simulink model "testemplanner_cs"  (R2023a)
settings: Solver=ode5  StartTime=0.0  StopTime=70  FixedStep=1/1000  RelTol=1e-3
PreLoadFcn:
  | mbxruntime.callbacks.PreLoadFcn(bdroot);
PostLoadFcn:
  | mbxruntime.callbacks.PostLoadFcn(bdroot);
InitFcn:
  | mbxruntime.callbacks.InitFcn(bdroot);
StartFcn:
  | mbxruntime.callbacks.StartFcn(bdroot);
StopFcn:
  | mbxruntime.callbacks.StopFcn(bdroot);
model workspace (MAT data in the model file):
  mbox_table : object (value not decoded)
  model_closed = 0
  sim_status = 0
values from neighbouring files (symbols this model uses):
  c_factor = 43.75    [emplanner_init.m]
  cf = -175016    [emplanner_init.m]
  cr = -130634    [emplanner_init.m]
  global_path_x = [-4.4795 -3.48011774493 -2.48199463442 -1.48514775065 -0.489582877207 0.504698358082 1.49769585569 2.48941007764 3.47984169183 4.46899144113 5.45686009523 6.44344843293 ... (3001 elements, 3001x1)]    [global_path.mat]
  global_path_y = [6.0531 6.0531 6.0531 6.0531 6.0531 6.0531 6.0531 6.0531 6.0531 6.0531 6.0531 6.0531 ... (3001 elements, 3001x1)]    [global_path.mat]
  KD_PID_distance = 0.0    (= 0)    [emplanner_init.m]
  KD_PID_speed = 0    [emplanner_init.m]
  KI_PID_distance = 0.0    (= 0)    [emplanner_init.m]
  KI_PID_speed = 0    [emplanner_init.m]
  KP_PID_distance = 0.5    [emplanner_init.m]
  KP_PID_speed = 1.8    [emplanner_init.m]
  la = 1.265    [emplanner_init.m]
  lb = 2.947-1.265    (= 1.682)    [emplanner_init.m]
  LQR_K1 = k(:,1)'    [emplanner_init.m]
  LQR_K2 = k(:,2)'    [emplanner_init.m]
  LQR_K3 = k(:,3)'    [emplanner_init.m]
  LQR_K4 = k(:,4)'    [emplanner_init.m]
  m = 2020    [emplanner_init.m]
  rack_displacement = [-39.14 , -37.2 , -35.29 , -33.43 , -31.6 , -29.81 , -28.06 , -26.34 , -24.66 ,      -23.01 , -21.38 , -19.79 , -18.23 , -16.69 , -15.18 , -13.7 , -12.23 , -10.8 , -9.38 , -7.98 ,     -6.61 , -5.25 , -3.91 , -2.59 , -1.29 , 0 , 1.27 , 2.54 , 3.78 , 5.02 , 6.24 , 7.46 , 8.66 ,      9.86 , 11.05 , 12.24 , 13.41 , 14.59 , 15.76 , 16.92 , 18.09 , 19.25 , 20.42 , 21.59 , 22.76 ,      23.93 , 25.11 , 26 ...(+26 chars)    [emplanner_init.m]
  right_wheel_ground = [-70 ,-67.2 , -64.4 , -61.6 , -58.8 , -56 , -53.2 , -50.4 , -47.6 , -44.8 , -42 ,      -39.2 , -36.4 , -33.6 , -30.8 , -28 , -25.2 , -22.4 , -19.6 , -16.8 , -14 , -11.2 , -8.4 , -5.6 ,      -2.8 , 0 , 2.8 , 5.6 , 8.4 , 11.2 , 14 , 16.8 , 19.6 , 22.4 , 25.2 , 28 , 30.8 , 33.6 , 36.4 ,      39.2 , 42 , 44.8 , 47.6 , 50.4 , 53.2 , 56 , 58.8 , 61.6 , 64.4 , 67.2 , 70 ]    [emplanner_init.m]
  vx_break_point = zeros(1,5000)    [emplanner_init.m]
undefined symbols (not defined in the file or in its folder): aubr, DiscIntNeverNeededParam, tablebr, vubr, warningInitialVelocity, x0
libraries: PreScanSimulinkLibrary x19, simulink x19, simulink_extras x6, Solver_SF x1
(part 8 of 10)

== matlab function testemplanner_cs/Audi_A8_Sedan_1/decision&planning module/EM Planner/cacul planning start gcs ==
  data: pre_trajectory_x input; planning_start_x output; pre_trajectory_y input; pre_trajectory_heading input; pre_trajectory_kappa input; pre_trajectory_speed input; pre_trajectory_accel input; pre_trajectory_time input; current_time input; host_x input; host_y input; host_heading_xy input; host_vx input; host_vy input; host_ax input; host_ay input; planning_start_y output; planning_start_heading output; planning_start_kappa output; planning_start_vx output; planning_start_vy output; planning_start_ax output; planning_start_ay output; planning_start_time output; stitch_x output; stitch_y output; stitch_heading output; stitch_kappa output; stitch_speed output; stitch_accel output; stitch_time output
function [planning_start_x, planning_start_y, planning_start_heading, planning_start_kappa, planning_start_vx, ...
    planning_start_vy, planning_start_ax, planning_start_ay, planning_start_time, stitch_x, stitch_y, stitch_heading, stitch_kappa, ...
    stitch_speed, stitch_accel, stitch_time] = fcn(pre_trajectory_x, pre_trajectory_y, pre_trajectory_heading, ...
    pre_trajectory_kappa, pre_trajectory_speed,  pre_trajectory_accel, pre_trajectory_time, current_time, host_x, ...
    host_y, host_heading_xy, host_vx, host_vy, host_ax, host_ay)


%该模块用来计算规划起点的信息：x,y,heading,kappa,vx,vy,ax,ay
%以及待拼接的轨迹信息：stitch_x,y,heading,kappa...
%输入参数：hostx,y,heading,kappa是世界坐标系下，而vx,vy,ax,ay是基于车辆坐标系
%输出参数：规划开始点以及待拼接轨迹的vx,vy,ax,ay都是基于世界坐标系
%stitch用来存储规划起点前20个点的轨迹，要生成缓冲矩阵

stitch_x = zeros(20,1);
stitch_y = zeros(20,1);
stitch_heading = zeros(20,1);
stitch_kappa = zeros(20,1);
stitch_speed = zeros(20,1);
stitch_accel = zeros(20,1);
%待拼接矩阵的时间序列，用-1代表无需拼接
stitch_time = ones(20,1)*-1;

%定义持久变量，若是第一次运行...
%若不是第一次运行...
persistent is_first_run
if isempty(is_first_run)
    is_first_run = 0;
    %第一次运行时没有上一周期的规划结果，可以根据车辆运动学模型递推出current_time+100ms时的状态
    %但第一次运行时，没有初始车速、加速度，也不需要轨迹拼接，直接拿定位信息当作规划起点即可
    planning_start_x = host_x; 
    planning_start_y = host_y;
    planning_start_heading = host_heading_xy;
    planning_start_kappa = 0;
    %下面这一行是老王的写法，有疑问
    % planning_start_kappa = 0;
    planning_start_vx = 0;
    planning_start_vy = 0;
    planning_start_ax = 0;
    planning_start_ay = 0;
    %planning_start_time为规划起点对应的时间戳，而不是规划开始的时间
    planning_start_time = current_time+0.1;

else
    %若不是第一次运行
    %首先要在上周期规划的轨迹中寻找current所对应的索引的信息（应该处在什么位置），根据实际所处位置做出判断控制的效果、是否需要拼接轨迹及规划起点
    for i = 1:length(pre_trajectory_time)-1
        if pre_trajectory_time(i) <= current_time && pre_trajectory_time(i+1) > current_time
            break;
        end
    end
    %遍历出的i即为current_time所对应的序号
    %根据定位位置与理想位置之间的误差判断是否需要轨迹拼接
    x_current = host_x;
    y_current = host_y;   
    heading_current = host_heading_xy;
    %kappa_current = 0; %老王的写法，为什么现在的曲率是0？
    kappa_current = 0;
    %定位的vxvy...是基于车辆坐标系的，要转换成世界坐标系
    vx_current = host_vx*cos(heading_current)-host_vy*sin(heading_current);
    vy_current = host_vy*cos(heading_current)+host_vx*sin(heading_current);
    ax_current = host_ax*cos(heading_current)-host_ay*sin(heading_current);
    ay_current = host_ay*cos(heading_current)+host_ax*sin(heading_current);
    x_desire = pre_trajectory_x(i);
    y_desire = pre_trajectory_y(i);
    heading_desire = pre_trajectory_heading(i);
    tor1 = [cos(heading_desire); sin(heading_desire)];
    nor1 = [-sin(heading_desire); cos(heading_desire)];
    %根据误差向量及切向量和法向量计算定位和理想位置间的横向误差及纵向误差
    err_vector = [x_current; y_current]-[x_desire; y_desire];
    %纵向误差
    err_long = abs(err_vector'*tor1);
    %侧向误差
    err_lat = abs(err_vector'*nor1);
    %规划的周期是100ms，即0.1s
    dt = 0.1;
    %判断控制是否跟上了轨迹,一般认为纵向误差大于2或者横向误差大于0.5时控制效果差
    if err_long > 2.5 || err_lat > 0.5
        %控制没有跟上轨迹，需要根据车辆运动学模型递推一个周期得到规划起点的状态,这里认为车辆在一个周期内做匀加速直线运动
        planning_start_x = x_current+vx_current*dt+0.5*ax_current*dt^2;
        planning_start_y = y_current+vy_current*dt+0.5*ay_current*dt^2;
        
        planning_start_kappa = kappa_current;
        planning_start_vx = vx_current+ax_current*dt;
        planning_start_vy = vy_current+ay_current*dt;
        planning_start_heading = atan2(planning_start_vy,planning_start_vx);
        planning_start_ax = ax_current;
        planning_start_ay = ay_current;
        %把planning_start_time（规划开始时间）表述为current_time+0.1是否不妥，规划开始时间应为current_time,此处仍有疑问
        planning_start_time = current_time+0.1;
        %控制没有跟上规划，递推出下个周期规划起点后再拿上周期的规划结果做轨迹拼接也就没有意义
    else
        %控制跟上了规划，需要做轨迹拼接
        %规划起点是current_time+0.1在时间戳里对应的索引对应的信息
        %先找到规划起点的索引
        for j = i:length(pre_trajectory_time)-1
            if pre_trajectory_time(j) <= current_time+0.1 && pre_trajectory_time(j+1) > current_time+0.1
                break;
            end
        end
        %j即为current_time+0.1在pre_trajectory_time时间戳里的索引
        planning_start_x = pre_trajectory_x(j);
        planning_start_y = pre_trajectory_y(j);
        %pre_trajecctory_speed,accel为轨迹的切向速度、加速度
        planning_start_heading = pre_trajectory_heading(j);
        planning_start_kappa = pre_trajectory_kappa(j);
        planning_start_vx = pre_trajectory_speed(j)*cos(planning_start_heading);
        planning_start_vy = pre_trajectory_speed(j)*sin(planning_start_heading);
        %加速度分为切向加速度和法向加速度
        %计算规划起点的切向量和法向量
        tor2 = [cos(planning_start_heading); sin(planning_start_heading)];
        nor2 = [-sin(planning_start_heading); cos(planning_start_heading)];
        %计算规划起点的切向加速度和法向加速度
        a_tor = pre_trajectory_accel(j)*tor2;
        a_nor = pre_trajectory_speed(j)^2*planning_start_kappa*nor2;
        planning_start_ax = a_tor(1)+a_nor(1);
        planning_start_ay = a_tor(2)+a_nor(2);
        %下面的规划开始时间同样有疑问
        % planning_start_time = pre_trajectory_time(j);  
        planning_start_time = current_time+0.1;

        %下面开始准备轨迹拼接，分为规划起点之前足够20个点和不足20个点两种情况
        if j > 20
            stitch_x = pre_trajectory_x(j-20:j-1);
            stitch_y = pre_trajectory_y(j-20:j-1);
            stitch_heading = pre_trajectory_heading(j-20:j-1);
            stitch_kappa = pre_trajectory_kappa(j-20:j-1);
            stitch_speed = pre_trajectory_speed(j-20:j-1);
            stitch_accel = pre_trajectory_accel(j-20:j-1);
            stitch_time = pre_trajectory_time(j-20:j-1);
        else
            %q:如果j=1怎么办？
            %a：只要i！=j，j就不会为1；即current_time的索引不能等于current_time+0.1的索引
            %轨迹点的采样要足够密集；eg:如果1s采样一个点，则会i=j...
            stitch_x(22-j:20) = pre_trajectory_x(1:j-1);
            stitch_y(22-j:20) = pre_trajectory_y(1:j-1);
            stitch_heading(22-j:20) = pre_trajectory_heading(1:j-1);
            stitch_kappa(22-j:20) = pre_trajectory_kappa(1:j-1);
            stitch_speed(22-j:20) = pre_trajectory_speed(1:j-1);
            stitch_accel(22-j:20) = pre_trajectory_accel(1:j-1);
            stitch_time(22-j:20) = pre_trajectory_time(1:j-1);
        end
    end

end

== matlab function testemplanner_cs/Audi_A8_Sedan_1/decision&planning module/referenceline provider/MATLAB Function4 ==
  data: path_x input; path_heading output; path_y input; path_kappa output
function [path_heading, path_kappa] = fcn(path_x, path_y)

%原理：heading=atan(dy/dx)
%kappa=dheading/ds
%ds=(dx^2+dy^2)^0.5
%但角度存在多值性问题，例如heading=atan(dy/dx)=heading+pi,在三角函数运算时会出现问题
%可以容忍heading+2pi（三角函数运算不会出现问题），但计算kappa=(dheading+2pi)/ds时要做特殊处理
%很多奇怪问题的根源就是角度的多值性处理不当
%中点欧拉法不能直接用

%dx,dy而不是角度用中点欧拉
dx = diff(path_x);
dy = diff(path_y);

dx_pre = [dx(1);dx];
dx_end = [dx;dx(end)];
dx_final = (dx_pre+dx_end)/2;

dy_pre = [dy(1);dy];
dy_end = [dy;dy(end)];
dy_final = (dy_pre+dy_end)/2;

%.^2是对每一个元素做平方运算，^2是矩阵运算
ds_final = sqrt(dx_final.^2+dy_final.^2);

%atan2为四象限反正切，将角度限定在-pi-pi
path_heading = atan2(dy_final,dx_final);

%对heading做差分，得到dheading，同样采用中点欧拉
dheading = diff(path_heading);
dheading_pre = [dheading(1);dheading];
dheading_after = [dheading;dheading(end)];
dheading_final = (dheading_pre+dheading_after)/2;

%认为dheading为很小量，用sin(dheading)近似代替heading,因为sin(dheading)与sin(dheading+2pi)相等
path_kappa = dheading_final./ds_final;

== matlab function testemplanner_cs/Audi_A8_Sedan_1/decision&planning module/EM Planner/match&proj point search2 ==
  data: match_point_index_set output; proj_x_set output; proj_y_set output; proj_heading_set output; proj_kappa_set output; x_set input; y_set input; frenet_x_set input; frenet_y_set input; frenet_heading_set input; frenet_kapppa_set input
function [match_point_index_set, proj_x_set, proj_y_set, proj_heading_set, proj_kappa_set] = fcn(x_set, y_set, frenet_x_set, frenet_y_set, ...
    frenet_heading_set, frenet_kapppa_set)

%待投影点是一个集合（自车，障碍物），每一个点分别遍历寻找匹配点，再寻找投影点
%匹配点集合要保存下来，作为下次遍历开始的起点
%第一次遍历，没有任何提示，从frenet点集第一点开始遍历
%若不是第一次遍历，从上次保存的匹配点开始，注意方向
%待投影点-寻找匹配点-寻找投影点-投影点（x,y,heading,kappa），保存匹配点索引集合

%（待）投影点数量未知，设置缓冲，最多批量处理128个点,信息冗余用NAN（not a number）处理
n = 128;
match_point_index_set = ones(n,1)*nan;
proj_x_set = ones(n,1)*nan;
proj_y_set = ones(n,1)*nan;
proj_heading_set = ones(n,1)*nan;
proj_kappa_set = ones(n,1)*nan;

%两种情况：第一次遍历，非第一次遍历
%声明两个全局变量，第一个用来判断是否初次运行，第二个用来存储上次匹配点集合
persistent is_first_run
persistent pre_match_point_index_set

if isempty(is_first_run)
    is_first_run = 0;
    pre_match_point_index_set = ones(n,1)*nan;
    %遍历每一个点寻找匹配点
    start_search_index = 1;
    for i = 1:length(x_set)
        if isnan(x_set(i))
            break;
        end
        increase_count = 0;
        min_distant = inf;
        for j = start_search_index:length(frenet_x_set)
            distant = (x_set(i)-frenet_x_set(j))^2+(y_set(i)-frenet_y_set(j))^2;
            if distant < min_distant
                min_distant = distant;
                increase_count = 0;
                match_point_index_set(i) = j;
            else
                increase_count = increase_count+1;
            end
            %第一次遍历连续增加50次停止
            if increase_count > 50
                break;
            end
        end
        %通过匹配点计算投影点
        %计算匹配点的位矢及方向向量
        vector_match_point = [frenet_x_set(match_point_index_set(i));frenet_y_set(match_point_index_set(i))];
        vector_match_point_direction = [cos(frenet_heading_set(match_point_index_set(i)));sin(frenet_heading_set(match_point_index_set(i)))];
        vector_d = [x_set(i);y_set(i)]-vector_match_point;
        ds = vector_d'*vector_match_point_direction;
        vector_ds = ds*vector_match_point_direction;
        vector_proj_point = vector_match_point+vector_ds;
        %计算投影点的x,y,heading,kappa
        proj_x_set(i) = vector_proj_point(1);
        proj_y_set(i) = vector_proj_point(2);
        proj_heading_set(i) = frenet_heading_set(match_point_index_set(i))+frenet_kapppa_set(match_point_index_set(i))*ds;
        proj_kappa_set(i) = frenet_kapppa_set(match_point_index_set(i));
    end
    pre_match_point_index_set = match_point_index_set;
else
    %如果不是第一次遍历
    for i = 1:length(x_set)

        if isnan(x_set(i))
            break;
        end
        %下面这行代码有严重问题，需要投影的不仅是自车，还有障碍物
        %而第一次运行时传感器可能监测不到障碍物，即算法会跳过is first run分支执行else分支
        %此时pre_match_point_index_set中除了自车都是nan，所以需要修复
        start_search_index = pre_match_point_index_set(i);
        increase_count_limit = 5;

        if isnan(start_search_index)
            %从第一个点开始遍历，并需要遍历50次防止取到局部极小值
            increase_count_limit = 50;
            start_search_index = 1;
        end

        increase_count = 0;
        min_distant = inf;
        %判断遍历方向
        vector_pre_match_point = [frenet_x_set(start_search_index);frenet_y_set(start_search_index)];
        vector_pre_match_point_direction = [cos(frenet_heading_set(start_search_index));sin(frenet_heading_set(start_search_index))];
        flag = ([x_set(i);y_set(i)]-vector_pre_match_point)'*vector_pre_match_point_direction;
        

        %正向遍历
        if flag > 0.001
            for j = start_search_index:length(frenet_x_set)
                distant = (x_set(i)-frenet_x_set(j))^2+(y_set(i)-frenet_y_set(j))^2;
                if distant < min_distant
                    min_distant = distant;
                    increase_count = 0;
                    match_point_index_set(i) = j;
                else
                    increase_count = increase_count+1;
                end
                %连续增加5次停止
                if increase_count > increase_count_limit
                    break;
                end
            end
            % %通过匹配点计算投影点
            % %计算匹配点的位矢及方向向量
            % vector_match_point = [frenet_x_set(match_point_index_set(i));frenet_y_set(match_point_index_set(i))];
            % vector_match_point_direction = [cos(frenet_heading_set(match_point_index_set(i)));sin(frenet_heading_set(match_point_index_set(i)))];
            % vector_d = [x_set(i);y_set(i)]-vector_match_point;
            % ds = vector_d'*vector_match_point_direction;
            % vector_ds = ds*vector_match_point_direction;
            % vector_proj_point = vector_match_point+vector_ds;
            % %计算投影点的x,y,heading,kappa
            % proj_x_set(i) = vector_proj_point(1);
            % proj_y_set(i) = vector_proj_point(2);
            % proj_heading_set(i) = frenet_heading_set(match_point_index_set(i))+frenet_kapppa_set(match_point_index_set(i))*ds;
            % proj_kappa_set(i) = frenet_kapppa_set(match_point_index_set(i));
        elseif flag < -0.001
            %反向遍历
             for j = start_search_index:-1:1
                distant = (x_set(i)-frenet_x_set(j))^2+(y_set(i)-frenet_y_set(j))^2;
                if distant < min_distant
                    min_distant = distant;
                    increase_count = 0;
                    match_point_index_set(i) = j;
                else
                    increase_count = increase_count+1;
                end
                %连续增加5次停止
                if increase_count > increase_count_limit
                    break;
                end
            end
        else
            match_point_index_set(i) = start_search_index;
        end

        %通过匹配点计算投影点
        %计算匹配点的位矢及方向向量
        vector_match_point = [frenet_x_set(match_point_index_set(i));frenet_y_set(match_point_index_set(i))];
        vector_match_point_direction = [cos(frenet_heading_set(match_point_index_set(i)));sin(frenet_heading_set(match_point_index_set(i)))];
        vector_d = [x_set(i);y_set(i)]-vector_match_point;
        ds = vector_d'*vector_match_point_direction;
        vector_ds = ds*vector_match_point_direction;
        vector_proj_point = vector_match_point+vector_ds;
        %计算投影点的x,y,heading,kappa
        proj_x_set(i) = vector_proj_point(1);
        proj_y_set(i) = vector_proj_point(2);
        proj_heading_set(i) = frenet_heading_set(match_point_index_set(i))+frenet_kapppa_set(match_point_index_set(i))*ds;
        proj_kappa_set(i) = frenet_kapppa_set(match_point_index_set(i));

    end
    pre_match_point_index_set = match_point_index_set;
end

== stateflow chart testemplanner_cs/Audi_A8_Sedan_1/Chart ==
  (default) -> (junction 5)
  (junction 5) -> (junction 7)
  (junction 7) -> (junction 9) [order 1] : [i >= 100]
  (junction 7) -> (junction 13) [order 2] : {
      | i = i+1;
      | }
  (junction 9) -> (junction 11) : {
      | do_planning;
      | i = 1;
      | }
  (junction 11) -> (junction 13)
  (junction 13) -> (junction 16)
  (junction 16) -> (junction 18) [order 1] : [j >= 10]
  (junction 16) -> (junction 22) [order 2] : {
      | j = j+1;
      | }
  (junction 18) -> (junction 20) : {
      | do_control;
      | j = 1;
      | }
  (junction 20) -> (junction 22)
  (junction 22) -> (junction 25)
  data: i local =1; j local =1
  events: do_planning output FUNCTION_CALL_EVENT; do_control output FUNCTION_CALL_EVENT

== matlab function testemplanner_cs/Audi_A8_Sedan_1/Perception Provider/MATLAB Function ==
  data: obs_x_set_gcs output; obs_y_set_gcs output; obs_velocity_set_gcs output; obs_heading_set_gcs output; host_x input; host_y input; host_xy_heading input; obs_range input; obs_theta input; obs_velocity input; obs_heading input
function [obs_x_set_gcs, obs_y_set_gcs, obs_velocity_set_gcs, obs_heading_set_gcs] = fcn(host_x, host_y, host_xy_heading, ...
    obs_range, obs_theta, obs_velocity, obs_heading)

%gcs为global coordinate system,即笛卡尔坐标系
%函数输入：
% host x定位在笛卡尔坐标系下的x坐标，host_y定位在笛卡尔坐标系下的y坐标，host_xy_heading:航向角
%obs_range:传感器到障碍物几何中心的距离，obs_theta:极坐标下坐标轴到range方向的角度
%obs_velocity:障碍物的绝对速度
%obs_heading:障碍物速度方向到坐标轴（N轴）的航向角
%输出：
% obs_xset_gcs:障碍物在笛卡尔坐标系下x坐标的集合
% obs_yset_gcs:....................y坐标.....
% obs_velocityset_gcs:.............速度......
% obs_headingset_gcs:..............速度的航向角的集合
% 注意坐标轴变换及单位变换，prescan输出的角度单位是rad

%传感器能识别最多32个障碍物，但事先不知道有多少障碍物，要做缓冲
obs_x_set_gcs = ones(32,1)*nan;
obs_y_set_gcs = ones(32,1)*nan;
obs_velocity_set_gcs = ones(32,1)*nan;
obs_heading_set_gcs = ones(32,1)*nan;

%在prescan的极坐标下顺时针为正，而我们认为逆时针为正
transfer_theta = -obs_theta.*pi/180;
transfer_velocity = obs_velocity;
transfer_heading = (90*ones(32,1)-obs_heading).*pi/180;
transfer_range_x = obs_range.*cos(transfer_theta+host_xy_heading);
transfer_range_y = obs_range.*sin(transfer_theta+host_xy_heading);

%计算障碍物在笛卡尔坐标系下的x,y,heading,velocity
%transfer_range是传感器到障碍物几何中心的距离，还需要考虑传感器到车辆中心的距离
%经过测算，传感器到车辆中心的距离大概是2.173
for i = 1:32
    %判断第i个障碍物是否存在
    if obs_range(i) ~= 0
        obs_x_set_gcs(i) = transfer_range_x(i)+host_x+2.173*cos(host_xy_heading);
        obs_y_set_gcs(i) = transfer_range_y(i)+host_y+2.173*sin(host_xy_heading);
        obs_velocity_set_gcs(i) = transfer_velocity(i);
        obs_heading_set_gcs(i) = transfer_heading(i);
    end
end

== matlab function testemplanner_cs/Audi_A8_Sedan_1/decision&planning module/EM Planner/generate index2s ==
  data: origin_match_point_index input; index2s output; origin_proj_x input; origin_proj_y input; path_x input; path_y input
function index2s = fcn(origin_match_point_index, origin_proj_x, origin_proj_y, path_x, path_y)

%该函数用来计算索引序号i对应的弧长s,对于每一个待投影的物体，都有一个匹配点（索引），index2s即为参考线原点到匹配点的弧长
%先计算索引点到参考线起始点的弧长
%再计算参考线起始点到自然坐标系原点（自车投影点）的弧长，作差得到frenet坐标系原点到索引点的弧长
%因为参考线有181个点，对应181个弧长(有一个点是坐标原点，该点到原点的距离认为是0)
n = 181;
index2s = zeros(n,1);
index2s(1) = 0;
for i = 2:n
    index2s(i) = sqrt((path_x(i)-path_x(i-1))^2+(path_y(i)-path_y(i-1))^2)+index2s(i-1);
end

%s0是一个通用函数，用来计算投影点到参考线原点的弧长(第一次调用时计算投影点到参考线起点的弧长)
s0 = CalcSFromIndex2s(index2s, origin_match_point_index, origin_proj_x, origin_proj_y, path_x, path_y);
index2s = index2s-ones(n,1)*s0;

end

%定义上述通用函数
function s0 = CalcSFromIndex2s(index2s, match_point_index, proj_x, proj_y, path_x, path_y)
%该函数第一次调用时用来计算自车投影点到参考线起点的弧长！！！
%该函数复用时用来计算障碍物投影点到参考线原点的弧长！！！
%我认为这里第一次使用与复用时的逻辑混乱，非常复杂

%我们要计算参考线起点到投影点（坐标系原点）的弧长
%并且已知参考线起点到匹配点的弧长index2s（i）
%所以要计算投影点与匹配点间的距离和相对位置关系
%向量的内积可以判断位置关系

%先定义投影点与匹配点的误差向量
vector1 = [proj_x; proj_y]-[path_x(match_point_index); path_y(match_point_index)];

%可以根据匹配点的临近点近似描述匹配点的方向向量
%1：如果匹配点前面还有点
%2：如果匹配点是最后一个点
if match_point_index < length(path_x)
    %定义匹配点的切向量
    vector2 = [path_x(match_point_index+1)-path_x(match_point_index); path_y(match_point_index+1)-path_y(match_point_index)];
else
    vector2 = [path_x(match_point_index)-path_x(match_point_index-1); path_y(match_point_index)-path_y(match_point_index-1)];
end

%判断匹配点与投影点的相对位置关系
%计算参考线起点到投影点的弧长
if vector1'*vector2 > 0
    %投影点在前，匹配点在后
    s0 = index2s(match_point_index)+sqrt(vector1'*vector1);
else
    %匹配点在前，投影点在后
    s0 = index2s(match_point_index)-sqrt(vector1'*vector1);
end
end

== matlab function testemplanner_cs/Audi_A8_Sedan_1/decision&planning module/EM Planner/Obs/match&proj point search2 ==
  data: match_point_index_set output; proj_x_set output; proj_y_set output; proj_heading_set output; proj_kappa_set output; x_set input; y_set input; frenet_x_set input; frenet_y_set input; frenet_heading_set input; frenet_kapppa_set input
function [match_point_index_set, proj_x_set, proj_y_set, proj_heading_set, proj_kappa_set] = fcn(x_set, y_set, frenet_x_set, frenet_y_set, ...
    frenet_heading_set, frenet_kapppa_set)

%待投影点是一个集合（自车，障碍物），每一个点分别遍历寻找匹配点，再寻找投影点
%匹配点集合要保存下来，作为下次遍历开始的起点
%第一次遍历，没有任何提示，从frenet点集第一点开始遍历
%若不是第一次遍历，从上次保存的匹配点开始，注意方向
%待投影点-寻找匹配点-寻找投影点-投影点（x,y,heading,kappa），保存匹配点索引集合

%（待）投影点数量未知，设置缓冲，最多批量处理128个点,信息冗余用NAN（not a number）处理
n = 128;
match_point_index_set = ones(n,1)*nan;
proj_x_set = ones(n,1)*nan;
proj_y_set = ones(n,1)*nan;
proj_heading_set = ones(n,1)*nan;
proj_kappa_set = ones(n,1)*nan;

%两种情况：第一次遍历，非第一次遍历
%声明两个全局变量，第一个用来判断是否初次运行，第二个用来存储上次匹配点集合
persistent is_first_run
persistent pre_match_point_index_set

if isempty(is_first_run)
    is_first_run = 0;
    pre_match_point_index_set = ones(n,1)*nan;
    %遍历每一个点寻找匹配点
    start_search_index = 1;
    for i = 1:length(x_set)
        if isnan(x_set(i))
            break;
        end
        increase_count = 0;
        min_distant = inf;
        for j = start_search_index:length(frenet_x_set)
            distant = (x_set(i)-frenet_x_set(j))^2+(y_set(i)-frenet_y_set(j))^2;
            if distant < min_distant
                min_distant = distant;
                increase_count = 0;
                match_point_index_set(i) = j;
            else
                increase_count = increase_count+1;
            end
            %第一次遍历连续增加50次停止
            if increase_count > 50
                break;
            end
        end
        %通过匹配点计算投影点
        %计算匹配点的位矢及方向向量
        vector_match_point = [frenet_x_set(match_point_index_set(i));frenet_y_set(match_point_index_set(i))];
        vector_match_point_direction = [cos(frenet_heading_set(match_point_index_set(i)));sin(frenet_heading_set(match_point_index_set(i)))];
        vector_d = [x_set(i);y_set(i)]-vector_match_point;
        ds = vector_d'*vector_match_point_direction;
        vector_ds = ds*vector_match_point_direction;
        vector_proj_point = vector_match_point+vector_ds;
        %计算投影点的x,y,heading,kappa
        proj_x_set(i) = vector_proj_point(1);
        proj_y_set(i) = vector_proj_point(2);
        proj_heading_set(i) = frenet_heading_set(match_point_index_set(i))+frenet_kapppa_set(match_point_index_set(i))*ds;
        proj_kappa_set(i) = frenet_kapppa_set(match_point_index_set(i));
    end
    pre_match_point_index_set = match_point_index_set;
else
    %如果不是第一次遍历
    for i = 1:length(x_set)

        if isnan(x_set(i))
            break;
        end
        %下面这行代码有严重问题，需要投影的不仅是自车，还有障碍物
        %而第一次运行时传感器可能监测不到障碍物，即算法会跳过is first run分支执行else分支
        %此时pre_match_point_index_set中除了自车都是nan，所以需要修复
        start_search_index = pre_match_point_index_set(i);
        increase_count_limit = 5;

        if isnan(start_search_index)
            %从第一个点开始遍历，并需要遍历50次防止取到局部极小值
            increase_count_limit = 50;
            start_search_index = 1;
        end

        increase_count = 0;
        min_distant = inf;
        %判断遍历方向
        vector_pre_match_point = [frenet_x_set(start_search_index);frenet_y_set(start_search_index)];
        vector_pre_match_point_direction = [cos(frenet_heading_set(start_search_index));sin(frenet_heading_set(start_search_index))];
        flag = ([x_set(i);y_set(i)]-vector_pre_match_point)'*vector_pre_match_point_direction;
        

        %正向遍历
        if flag > 0.001
            for j = start_search_index:length(frenet_x_set)
                distant = (x_set(i)-frenet_x_set(j))^2+(y_set(i)-frenet_y_set(j))^2;
                if distant < min_distant
                    min_distant = distant;
                    increase_count = 0;
                    match_point_index_set(i) = j;
                else
                    increase_count = increase_count+1;
                end
                %连续增加5次停止
                if increase_count > increase_count_limit
                    break;
                end
            end
            % %通过匹配点计算投影点
            % %计算匹配点的位矢及方向向量
            % vector_match_point = [frenet_x_set(match_point_index_set(i));frenet_y_set(match_point_index_set(i))];
            % vector_match_point_direction = [cos(frenet_heading_set(match_point_index_set(i)));sin(frenet_heading_set(match_point_index_set(i)))];
            % vector_d = [x_set(i);y_set(i)]-vector_match_point;
            % ds = vector_d'*vector_match_point_direction;
            % vector_ds = ds*vector_match_point_direction;
            % vector_proj_point = vector_match_point+vector_ds;
            % %计算投影点的x,y,heading,kappa
            % proj_x_set(i) = vector_proj_point(1);
            % proj_y_set(i) = vector_proj_point(2);
            % proj_heading_set(i) = frenet_heading_set(match_point_index_set(i))+frenet_kapppa_set(match_point_index_set(i))*ds;
            % proj_kappa_set(i) = frenet_kapppa_set(match_point_index_set(i));
        elseif flag < -0.001
            %反向遍历
             for j = start_search_index:-1:1
                distant = (x_set(i)-frenet_x_set(j))^2+(y_set(i)-frenet_y_set(j))^2;
                if distant < min_distant
                    min_distant = distant;
                    increase_count = 0;
                    match_point_index_set(i) = j;
                else
                    increase_count = increase_count+1;
                end
                %连续增加5次停止
                if increase_count > increase_count_limit
                    break;
                end
            end
        else
            match_point_index_set(i) = start_search_index;
        end

        %通过匹配点计算投影点
        %计算匹配点的位矢及方向向量
        vector_match_point = [frenet_x_set(match_point_index_set(i));frenet_y_set(match_point_index_set(i))];
        vector_match_point_direction = [cos(frenet_heading_set(match_point_index_set(i)));sin(frenet_heading_set(match_point_index_set(i)))];
        vector_d = [x_set(i);y_set(i)]-vector_match_point;
        ds = vector_d'*vector_match_point_direction;
        vector_ds = ds*vector_match_point_direction;
        vector_proj_point = vector_match_point+vector_ds;
        %计算投影点的x,y,heading,kappa
        proj_x_set(i) = vector_proj_point(1);
        proj_y_set(i) = vector_proj_point(2);
        proj_heading_set(i) = frenet_heading_set(match_point_index_set(i))+frenet_kapppa_set(match_point_index_set(i))*ds;
        proj_kappa_set(i) = frenet_kapppa_set(match_point_index_set(i));

    end
    pre_match_point_index_set = match_point_index_set;
end

== matlab function testemplanner_cs/Audi_A8_Sedan_1/decision&planning module/EM Planner/Cartesian2Frenet-panning start point/S&L calcu ==
  data: s_set output; l_set output; x_set input; y_set input; proj_x_set input; proj_y_set input; proj_heading_set input; index2s input; planning_start_match_point_index input; frenet_x input; frenet_y input
function [s_set, l_set] = fcn(x_set, y_set, proj_x_set, proj_y_set, proj_heading_set, index2s, ...
    planning_start_match_point_index, frenet_x, frenet_y)

%此函数用来存储规划起点及障碍物在以自车定位的投影点为参考线原点的frenet坐标系的sl坐标
%由于不知道规划起点及障碍物共多少个，故需要缓冲
%计算s时直接复用index2s模块中写好的子函数
%共有128个点

n = 128;
s_set = ones(n,1)*nan;
l_set = ones(n,1)*nan;
 
for i = 1:length(x_set)
    if isnan(x_set(i))
        break;
    end
    %计算规划起点或障碍物的匹配点到参考线原点(自车在参考线上的投影点)的弧长
    s_set(i) = CalcSFromIndex2s(index2s, planning_start_match_point_index, proj_x_set(i), proj_y_set(i), frenet_x, frenet_y);
    vector_rh = [x_set(i); y_set(i)];
    vector_rr = [proj_x_set(i); proj_y_set(i)];
    vector_nor_r = [-sin(proj_heading_set(i)); cos(proj_heading_set(i))];
    l_set(i) = (vector_rh-vector_rr)'*vector_nor_r;
end
end

%复用index2s中写好的计算弧长s的子函数
function s0 = CalcSFromIndex2s(index2s, match_point_index, proj_x, proj_y, path_x, path_y)
%该函数第一次调用时用来计算自车投影点到参考线起点的弧长！！！
%该函数复用时用来计算障碍物投影点到参考线原点的弧长！！！
%我认为这里第一次使用与复用时的逻辑混乱，非常复杂

%我们要计算参考线起点到投影点（坐标系原点）的弧长
%并且已知参考线起点到匹配点的弧长index2s（i）
%所以要计算投影点与匹配点间的距离和相对位置关系
%向量的内积可以判断位置关系

%先定义投影点与匹配点的误差向量
vector1 = [proj_x; proj_y]-[path_x(match_point_index); path_y(match_point_index)];

%可以根据匹配点的临近点近似描述匹配点的方向向量
%1：如果匹配点前面还有点
%2：如果匹配点是最后一个点
if match_point_index < length(path_x)
    %定义匹配点的切向量
    vector2 = [path_x(match_point_index+1)-path_x(match_point_index); path_y(match_point_index+1)-path_y(match_point_index)];
else
    vector2 = [path_x(match_point_index)-path_x(match_point_index-1); path_y(match_point_index)-path_y(match_point_index-1)];
end

%判断匹配点与投影点的相对位置关系
%计算参考线起点到投影点的弧长
if vector1'*vector2 > 0
    %投影点在前，匹配点在后
    s0 = index2s(match_point_index)+sqrt(vector1'*vector1);
else
    %匹配点在前，投影点在后
    s0 = index2s(match_point_index)-sqrt(vector1'*vector1);
end
end

== matlab function testemplanner_cs/Audi_A8_Sedan_1/decision&planning module/EM Planner/Cartesian2Frenet-panning start point/S_dot&L_dot&dL calcu  ==
  data: s_dot_set output; vx_set input; vy_set input; proj_heading_set input; proj_kappa_set input; l_set input; l_dot_set output; dl_set output
function [s_dot_set, l_dot_set, dl_set]  = fcn(vx_set, vy_set, proj_heading_set, proj_kappa_set, l_set)

%这个函数用来存储s_dot&l_dot&dl的集合
n = 128;
s_dot_set = ones(n,1)*nan;
l_dot_set = ones(n,1)*nan;
dl_set = ones(n,1)*nan;

for i = 1:length(l_set)
    if isnan(l_set(i))
        break;
    end
    vector_vh = [vx_set(i); vy_set(i)];
    vector_tor_r = [cos(proj_heading_set(i)); sin(proj_heading_set(i))];
    vector_nor_r = [-sin(proj_heading_set(i)); cos(proj_heading_set(i))];
    s_dot_set(i) = vector_vh'*vector_tor_r/(1-proj_kappa_set(i)*l_set(i));
    l_dot_set(i) = vector_vh'*vector_nor_r;

    %dl=l_dot/s_dot,所以s_dot不能为0，这里要打一个补丁，当s_dot趋于0时，dl=0
    if abs(s_dot_set(i)) < 1e-6
        dl_set(i) = 0;
    else
        dl_set(i) = l_dot_set(i)/s_dot_set(i);
    end

end

end

== matlab function testemplanner_cs/Audi_A8_Sedan_1/decision&planning module/EM Planner/Cartesian2Frenet-panning start point/S_dot2&L_dot2&ddL calcu ==
  data: ax_set input; s_dot2_set output; ay_set input; proj_heading_set input; proj_kappa_set input; l_set input; dl_set input; s_dot_set input; l_dot2_set output; ddl_set output
function [s_dot2_set, l_dot2_set, ddl_set] = fcn(ax_set, ay_set, proj_heading_set, proj_kappa_set, l_set, dl_set...
    , s_dot_set)

%该函数用来存储s_dot2&l_dot2&ddl,同样要设置缓冲
n = 128;
s_dot2_set = ones(n,1)*nan;
l_dot2_set = ones(n,1)*nan; 
ddl_set = ones(n,1)*nan;

for i = 1:length(l_set)
    if isnan(l_set(i))
        break;
    end
    vector_ah = [ax_set(i); ay_set(i)];
    vector_tor_r = [cos(proj_heading_set(i)); sin(proj_heading_set(i))];
    vector_nor_r = [-sin(proj_heading_set(i)); cos(proj_heading_set(i))];

    %kr'=dkr/ds,曲率随弧长的变化速率很小，kr'=0
    s_dot2_set(i) = vector_ah'*vector_tor_r/(1-proj_kappa_set(i)*l_set(i))+proj_kappa_set(i)*dl_set(i)*s_dot_set(i)^2/(1-proj_kappa_set(i)*l_set(i))...
        +s_dot_set(i)^2*proj_kappa_set(i)*dl_set(i)/(1-proj_kappa_set(i)*l_set(i));

    l_dot2_set(i) = vector_ah'*vector_nor_r-proj_kappa_set(i)*s_dot_set(i)^2*(1-proj_kappa_set(i)*l_set(i));

    %ddl的表达式分母上有s_dot,同样要确保s_dot不为0
    if abs(s_dot_set(i)) < 1e-6
        ddl_set(i) = 0;
    else
        ddl_set(i) = (l_dot2_set(i)-dl_set(i)*s_dot2_set(i))/s_dot_set(i)^2; 
    end

end

end

== matlab function testemplanner_cs/Audi_A8_Sedan_1/decision&planning module/EM Planner/Obs/Obs Filter ==
  data: host_x input; obs_x_final_set output; host_y input; obs_x_set_gcs input; obs_y_set_gcs input; obs_velocity_set_gcs input; obs_heading_set_gcs input; host_heading_xy input; obs_y_final_set output; obs_velocity_final_set output; obs_heading_final_set output
function [obs_x_final_set, obs_y_final_set, obs_velocity_final_set, obs_heading_final_set] = fcn(host_x, host_y, obs_x_set_gcs, ...
    obs_y_set_gcs, obs_velocity_set_gcs, obs_heading_set_gcs, host_heading_xy)

%该函数用来筛选范围内的障碍物（包括静态和动态）
%筛选纵向-10：60，横向-10：10范围内单车道上的障碍物
%完全体的EMPLANNER是多车道并行计算
%传感器最多识别32个障碍物，需要设置缓冲

n = 32;
obs_x_final_set = ones(n,1)*nan;
obs_y_final_set = ones(n,1)*nan;
obs_velocity_final_set = ones(n,1)*nan;
obs_heading_final_set = ones(n,1)*nan;
count = 1;

%通过障碍物与自车间的距离判断
for i = 1:length(obs_x_set_gcs)
    if isnan(obs_x_set_gcs(i))
        break;
    end
    vector_err = [obs_x_set_gcs(i); obs_y_set_gcs(i)]-[host_x; host_y];
    vector_tor_h = [cos(host_heading_xy); sin(host_heading_xy)];
    vector_nor_h = [-sin(host_heading_xy); cos(host_heading_xy)];
    %车身坐标系下的纵向距离及横向距离
    distant_long = vector_err'*vector_tor_h;
    distant_later = vector_err'*vector_nor_h;

    if distant_long < 60 && distant_long > -10 && distant_later > -10 && distant_later < 10
        obs_x_final_set(count) = obs_x_set_gcs(i);
        obs_y_final_set(count) = obs_y_set_gcs(i);
        obs_velocity_final_set(count) = obs_velocity_set_gcs(i);
        obs_heading_final_set(count) = obs_heading_set_gcs(i);
        count = count+1;
    end
end



end

== matlab function testemplanner_cs/Audi_A8_Sedan_1/decision&planning module/EM Planner/Obs/Static&Dynamic Obs Filter ==
  data: obs_x_final_set input; static_obs_x_set output; obs_y_final_set input; obs_velocity_final_set input; obs_heading_final_set input; static_obs_y_set output; dynamic_obs_x_set output; dynamic_obs_y_set output; dynamic_obs_vx_set output; dynamic_obs_vy_set output
function [static_obs_x_set, static_obs_y_set, ...
    dynamic_obs_x_set, dynamic_obs_y_set, dynamic_obs_vx_set, dynamic_obs_vy_set] = fcn(...
    obs_x_final_set, obs_y_final_set, obs_velocity_final_set, obs_heading_final_set)

%该函数的作用是把范围内的静/动态障碍物分离开来
%根据障碍物速度的大小作为判断障碍物静动态的准则
%还是要做缓冲

n = 32;
static_obs_x_set = ones(n,1)*nan;
static_obs_y_set = ones(n,1)*nan;
% static_obs_velocity_set = ones(n,1)*nan;
% static_obs_heading_set = ones(n,1)*nan;
dynamic_obs_x_set = ones(n,1)*nan;
dynamic_obs_y_set = ones(n,1)*nan;
dynamic_obs_vx_set = ones(n,1)*nan;
dynamic_obs_vy_set = ones(n,1)*nan;
static_count = 1;
dynamic_count = 1;

for i = 1:length(obs_x_final_set)
    if isnan(obs_x_final_set(i))
        break;
    end
    if abs(obs_velocity_final_set(i)) < 0.1
        %属于静态障碍物
        static_obs_x_set(static_count) = obs_x_final_set(i);
        static_obs_y_set(static_count) = obs_y_final_set(i);
        % static_obs_velocity_set(static_count) = obs_velocity_final_set(i);
        % static_obs_heading_set(static_count) = obs_heading_final_set(i);
        static_count = static_count+1;
    else
        %属于动态障碍物
        dynamic_obs_x_set(dynamic_count) = obs_x_final_set(i);
        dynamic_obs_y_set(dynamic_count) = obs_y_final_set(i);
        % dynamic_obs_velocity_set(dynamic_count) = obs_velocity_final_set(i);
        % dynamic_obs_heading_set(dynamic_count) = obs_heading_final_set(i);
        dynamic_count = dynamic_count+1;
    end
end





end

== matlab function testemplanner_cs/Audi_A8_Sedan_1/control module/control main/longitudinal control double PID/MATLAB Function1 ==
  data: u input; throttle output; brake output
function [throttle,brake] = fcn(u)
    if u>=0
        throttle=u;
        brake=0;
    else
        throttle=0;
        brake=-u;
    end

== matlab function testemplanner_cs/Audi_A8_Sedan_1/decision&planning module/EM Planner/MATLAB Function1 ==
  data: s input; l input
function fcn(s, l)

coder.extrinsic("plot")
plot(s, l)

== matlab function testemplanner_cs/Audi_A8_Sedan_1/control module/control main/lateral control LQR/err_kappa_calculate_module ==
  data: x input; y input; phi input; vx input; vy input; phi_dot input; xr input; yr input; thetar input; kappar input; err output; es output; s_dot output
function [err,es,s_dot] = fcn(x,y,phi,vx,vy,phi_dot,xr,yr,thetar,kappar)
    
    tor=[cos(thetar);sin(thetar)];
    nor=[-sin(thetar);cos(thetar)];
    d_err=[x-xr;y-yr];
    ed=nor'*d_err;
    es=tor'*d_err;
    %projection_point_thetar=thetar(dmin);%apollo
    projection_point_thetar=thetar+kappar*es;
    ed_dot=vy*cos(phi-projection_point_thetar)+vx*sin(phi-projection_point_thetar);
    %%%%%%%%%
    ephi=sin(phi-projection_point_thetar);
    %%%%%%%%%
    ss_dot=vx*cos(phi-projection_point_thetar)-vy*sin(phi-projection_point_thetar);
    s_dot=ss_dot/(1-kappar*ed);
    ephi_dot=phi_dot-kappar*s_dot;
    err=[ed;ed_dot;ephi;ephi_dot];
    
    
    
    
    
    
    
    
    
    
    
    


end

== matlab function testemplanner_cs/Audi_A8_Sedan_1/control module/control main/lateral control LQR/feed_forword_control ==
  data: vx input; a input; forword_angle output; b input; m input; cf input; cr input; k input; kr input
function forword_angle = fcn(vx,a,b,m,cf,cr,k,kr)
    forword_angle=kr*(a+b-b*k(3)-(m*vx*vx/(a+b))*((b/cf)+(a/cr)*k(3)-(a/cr)));
end

== matlab function testemplanner_cs/Audi_A8_Sedan_1/control module/control main/lateral control LQR/feedback_control+feedforword_control ==
  data: k input; angle output; err input; forword_angle input
function angle = fcn(k,err,forword_angle)

    angle=-k*err+forword_angle;
end

== matlab function testemplanner_cs/Audi_A8_Sedan_1/control module/control main/lateral control LQR/calc lqr K ==
  data: k1 input; k output; k2 input; k3 input; k4 input; vx input
function k  = fcn(k1,k2,k3,k4,vx)
    if abs(vx)<0.1
        k=[0,0,0,0];
    else
       
        k=[k1,k2,k3,k4];
    end
end

== matlab function testemplanner_cs/Audi_A8_Sedan_1/control module/control main/lateral control LQR/predict_module ==
  data: x input; pred_x_ctrl output; y input; phi input; vx input; vy input; phi_dot input; ts input; pred_y_ctrl output; pred_yaw_ctrl output; pred_vx_ctrl output; pred_vy_ctrl output; pred_yaw_dot_ctrl output
function [pred_x_ctrl,pred_y_ctrl,pred_yaw_ctrl,pred_vx_ctrl,pred_vy_ctrl,pred_yaw_dot_ctrl] = fcn(x,y,phi,vx,vy,phi_dot,ts)
    pred_x_ctrl=x+vx*ts*cos(phi)-vy*ts*sin(phi);
    pred_y_ctrl=y+vy*ts*cos(phi)+vx*ts*sin(phi);
    pred_yaw_ctrl=phi;
    pred_vx_ctrl=vx;
    pred_vy_ctrl=vy;
    pred_yaw_dot_ctrl=phi_dot;
end

== matlab function testemplanner_cs/Audi_A8_Sedan_1/decision&planning module/EM Planner/Obs/Cartesian2Frenet-static obs/S&L calcu ==
  data: s_set output; l_set output; x_set input; y_set input; proj_x_set input; proj_y_set input; proj_heading_set input; index2s input; planning_start_match_point_index input; frenet_x input; frenet_y input
function [s_set, l_set] = fcn(x_set, y_set, proj_x_set, proj_y_set, proj_heading_set, index2s, ...
    planning_start_match_point_index, frenet_x, frenet_y)

%此函数用来存储规划起点及障碍物在以自车定位的投影点为参考线原点的frenet坐标系的sl坐标
%由于不知道规划起点及障碍物共多少个，故需要缓冲
%计算s时直接复用index2s模块中写好的子函数
%共有128个点

n = 128;
s_set = ones(n,1)*nan;
l_set = ones(n,1)*nan;
 
for i = 1:length(x_set)
    if isnan(x_set(i))
        break;
    end
    %计算规划起点或障碍物的匹配点到参考线原点(自车在参考线上的投影点)的弧长
    s_set(i) = CalcSFromIndex2s(index2s, planning_start_match_point_index(i), proj_x_set(i), proj_y_set(i), frenet_x, frenet_y);
    vector_rh = [x_set(i); y_set(i)];
    vector_rr = [proj_x_set(i); proj_y_set(i)];
    vector_nor_r = [-sin(proj_heading_set(i)); cos(proj_heading_set(i))];
    l_set(i) = (vector_rh-vector_rr)'*vector_nor_r;
end
end

%复用index2s中写好的计算弧长s的子函数
function s0 = CalcSFromIndex2s(index2s, match_point_index, proj_x, proj_y, path_x, path_y)
%该函数第一次调用时用来计算自车投影点到参考线起点的弧长！！！
%该函数复用时用来计算障碍物投影点到参考线原点的弧长！！！
%我认为这里第一次使用与复用时的逻辑混乱，非常复杂

%我们要计算参考线起点到投影点（坐标系原点）的弧长
%并且已知参考线起点到匹配点的弧长index2s（i）
%所以要计算投影点与匹配点间的距离和相对位置关系
%向量的内积可以判断位置关系

%先定义投影点与匹配点的误差向量
vector1 = [proj_x; proj_y]-[path_x(match_point_index); path_y(match_point_index)];

%可以根据匹配点的临近点近似描述匹配点的方向向量
%1：如果匹配点前面还有点
%2：如果匹配点是最后一个点
if match_point_index < length(path_x)
    %定义匹配点的切向量
    vector2 = [path_x(match_point_index+1)-path_x(match_point_index); path_y(match_point_index+1)-path_y(match_point_index)];
else
    vector2 = [path_x(match_point_index)-path_x(match_point_index-1); path_y(match_point_index)-path_y(match_point_index-1)];
end

%判断匹配点与投影点的相对位置关系
%计算参考线起点到投影点的弧长
if vector1'*vector2 > 0
    %投影点在前，匹配点在后
    s0 = index2s(match_point_index)+sqrt(vector1'*vector1);
else
    %匹配点在前，投影点在后
    s0 = index2s(match_point_index)-sqrt(vector1'*vector1);
end
end

== matlab function testemplanner_cs/Audi_A8_Sedan_1/control module/control main/chassic steering system/MATLAB Function ==
  data: u input; right_steer output; la input; lb input
function right_steer = fcn(u,la,lb)
if abs(u)<1e-2
   right_steer = u;
else
   R =  (la+lb)/tan(u);
   right_steer = atan((la+lb)/(R+1.624/2));
end

== matlab function testemplanner_cs/Audi_A8_Sedan_1/decision&planning module/EM Planner/Obs/Cartesian2Frenet-static obs/S_dot&L_dot&dL calcu  ==
  data: s_dot_set output; vx_set input; vy_set input; proj_heading_set input; proj_kappa_set input; l_set input; l_dot_set output; dl_set output
function [s_dot_set, l_dot_set, dl_set]  = fcn(vx_set, vy_set, proj_heading_set, proj_kappa_set, l_set)

%这个函数用来存储s_dot&l_dot&dl的集合
n = 128;
s_dot_set = ones(n,1)*nan;
l_dot_set = ones(n,1)*nan;
dl_set = ones(n,1)*nan;

for i = 1:length(l_set)
    if isnan(l_set(i))
        break;
    end
    vector_vh = [vx_set(i); vy_set(i)];
    vector_tor_r = [cos(proj_heading_set(i)); sin(proj_heading_set(i))];
    vector_nor_r = [-sin(proj_heading_set(i)); cos(proj_heading_set(i))];
    s_dot_set(i) = vector_vh'*vector_tor_r/(1-proj_kappa_set(i)*l_set(i));
    l_dot_set(i) = vector_vh'*vector_nor_r;

    %dl=l_dot/s_dot,所以s_dot不能为0，这里要打一个补丁，当s_dot趋于0时，dl=0
    if abs(s_dot_set(i)) < 1e-6
        dl_set(i) = 0;
    else
        dl_set(i) = l_dot_set(i)/s_dot_set(i);
    end

end

end

== matlab function testemplanner_cs/Audi_A8_Sedan_1/decision&planning module/EM Planner/Obs/Cartesian2Frenet-static obs/S_dot2&L_dot2&ddL calcu ==
  data: ax_set input; s_dot2_set output; ay_set input; proj_heading_set input; proj_kappa_set input; l_set input; dl_set input; s_dot_set input; l_dot2_set output; ddl_set output
function [s_dot2_set, l_dot2_set, ddl_set] = fcn(ax_set, ay_set, proj_heading_set, proj_kappa_set, l_set, dl_set...
    , s_dot_set)

%该函数用来存储s_dot2&l_dot2&ddl,同样要设置缓冲
n = 128;
s_dot2_set = ones(n,1)*nan;
l_dot2_set = ones(n,1)*nan; 
ddl_set = ones(n,1)*nan;

for i = 1:length(l_set)
    if isnan(l_set(i))
        break;
    end
    vector_ah = [ax_set(i); ay_set(i)];
    vector_tor_r = [cos(proj_heading_set(i)); sin(proj_heading_set(i))];
    vector_nor_r = [-sin(proj_heading_set(i)); cos(proj_heading_set(i))];

    %kr'=dkr/ds,曲率随弧长的变化速率很小，kr'=0
    s_dot2_set(i) = vector_ah'*vector_tor_r/(1-proj_kappa_set(i)*l_set(i))+proj_kappa_set(i)*dl_set(i)*s_dot_set(i)^2/(1-proj_kappa_set(i)*l_set(i))...
        +s_dot_set(i)^2*proj_kappa_set(i)*dl_set(i)/(1-proj_kappa_set(i)*l_set(i));

    l_dot2_set(i) = vector_ah'*vector_nor_r-proj_kappa_set(i)*s_dot_set(i)^2*(1-proj_kappa_set(i)*l_set(i));

    %ddl的表达式分母上有s_dot,同样要确保s_dot不为0
    if abs(s_dot_set(i)) < 1e-6
        ddl_set(i) = 0;
    else
        ddl_set(i) = (l_dot2_set(i)-dl_set(i)*s_dot2_set(i))/s_dot_set(i)^2; 
    end

end

end
